simulink model "ObserverStatesPlusPert"  (R2022b)
settings: Solver=ode5  StartTime=0.0  StopTime=10  FixedStep=0.001  RelTol=1e-3
InitFcn:
  | ObsStatesPlusPertParameters
values from neighbouring files (symbols this model uses):
  A = 0.40648    [ObsStatesPlusPertParameters.m]
  a1 = e1/e2    (= 1.03595661896)    [ObsStatesPlusPertParameters.m]
  a2 = f2/e2    (= 0.828055342045)    [ObsStatesPlusPertParameters.m]
  a3 = f1/e2    (= 0.221523633506)    [ObsStatesPlusPertParameters.m]
  a4 = g2/e2    (= 0.768639508071)    [ObsStatesPlusPertParameters.m]
  a5 = g1/e2    (= 0.205628546835)    [ObsStatesPlusPertParameters.m]
  ax = 10.2    [ObsStatesPlusPertParameters.m]
  B = 0.40648    [ObsStatesPlusPertParameters.m]
  baralpha1 = 8    [ObsStatesPlusPertParameters.m]
  barbeta = 12.5    [ObsStatesPlusPertParameters.m]
  C = [1 , 0]    [ObsStatesPlusPertParameters.m]
  Cbar = [1, 0, 0]    [ObsStatesPlusPertParameters.m]
  G = 0.00833    [ObsStatesPlusPertParameters.m]
  Gamma = [ -a1, -a5 ... (first row only)    [ObsStatesPlusPertParameters.m]
  Gamma_bar = [    0,    ax,   0 ... (first row only)    [ObsStatesPlusPertParameters.m]
  k1 = 120    [ObsStatesPlusPertParameters.m]
  k1_pi = 20    [ObsStatesPlusPertParameters.m]
  k2 = 100    [ObsStatesPlusPertParameters.m]
  k2_pi = 1.3    [ObsStatesPlusPertParameters.m]
  kappa = 0.09    [ObsStatesPlusPertParameters.m]
  kobs = lobs/2 - (theta^3)/(2*ax)    (= 66.5945098039)    [ObsStatesPlusPertParameters.m]
  l = 0.65    [ObsStatesPlusPertParameters.m]
  L_b = 15    [ObsStatesPlusPertParameters.m]
  L_p = 7    [ObsStatesPlusPertParameters.m]
  M_b = 16    [ObsStatesPlusPertParameters.m]
  M_p = 7.1    [ObsStatesPlusPertParameters.m]
  omega = 1    [ObsStatesPlusPertParameters.m]
  Sinv = [    3*theta                            ,    3*((theta^2)/(ax))                     ,   (1/(ax))*(theta^3 + 2*kobs*ax) ... (first row only)    [ObsStatesPlusPertParameters.m]
settings Model: Creator=CIO  LastModifiedBy=gerar

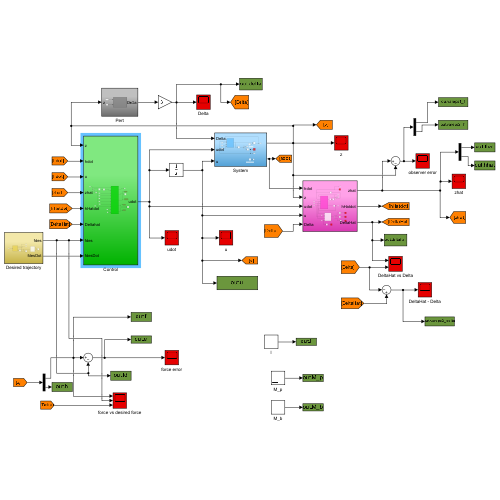
[thumbnail: Simulink's stored preview of the top-level diagram]
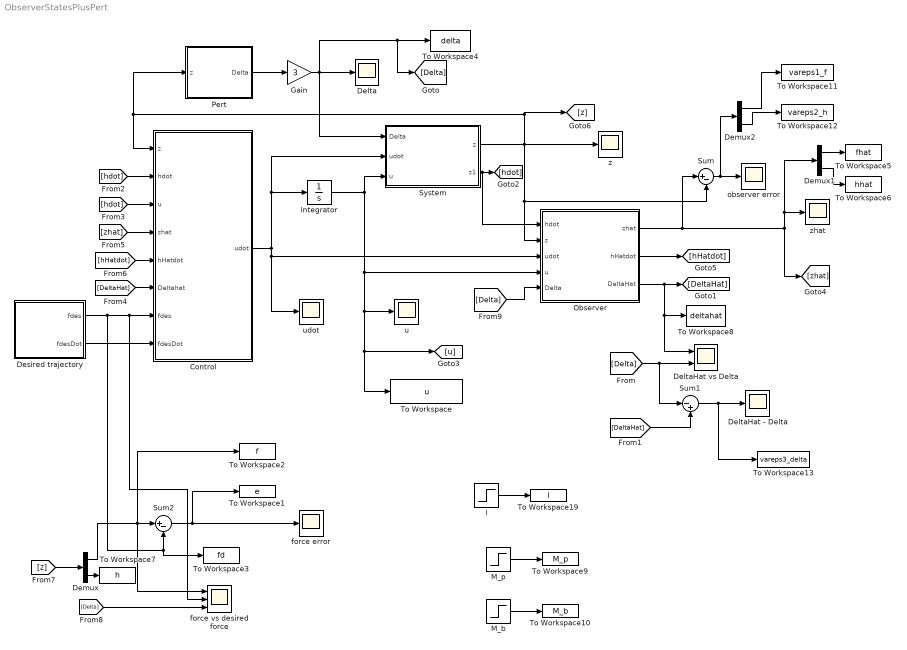
== system ObserverStatesPlusPert ==
  Control : Subsystem
  Delta : Scope
  DeltaHat - Delta : Scope
  DeltaHat vs Delta : Scope  NumInputPorts=2
  Demux : Demux  Outputs=2
  Demux1 : Demux  Outputs=2
  Demux2 : Demux  Outputs=2
  Desired trajectory : Subsystem
  Gain : Gain  Gain=3
  Integrator : Integrator
  M_b : Step  Time=0  Before=M_b  After=M_b  SampleTime=0
  M_p : Step  Time=0  Before=M_p  After=M_p  SampleTime=0
  Observer : Subsystem
  Pert : Subsystem
  Sum : Sum  Inputs=|+-
  Sum1 : Sum  Inputs=|-+
  Sum2 : Sum  Inputs=|+-
  System : Subsystem
  To Workspace : ToWorkspace  VariableName=u  SaveFormat=Timeseries  SampleTime=-1
  To Workspace1 : ToWorkspace  VariableName=e  SaveFormat=Timeseries  SampleTime=-1
  To Workspace10 : ToWorkspace  VariableName=M_b  SaveFormat=Timeseries  SampleTime=-1
  To Workspace11 : ToWorkspace  VariableName=vareps1_f  SaveFormat=Timeseries  SampleTime=-1
  To Workspace12 : ToWorkspace  VariableName=vareps2_h  SaveFormat=Timeseries  SampleTime=-1
  To Workspace13 : ToWorkspace  VariableName=vareps3_delta  SaveFormat=Timeseries  SampleTime=-1
  To Workspace19 : ToWorkspace  VariableName=l  SaveFormat=Timeseries  SampleTime=-1
  To Workspace2 : ToWorkspace  VariableName=f  SaveFormat=Timeseries  SampleTime=-1
  To Workspace3 : ToWorkspace  VariableName=fd  SaveFormat=Timeseries  SampleTime=-1
  To Workspace4 : ToWorkspace  VariableName=delta  SaveFormat=Timeseries  SampleTime=-1
  To Workspace5 : ToWorkspace  VariableName=fhat  SaveFormat=Timeseries  SampleTime=-1
  To Workspace6 : ToWorkspace  VariableName=hhat  SaveFormat=Timeseries  SampleTime=-1
  To Workspace7 : ToWorkspace  VariableName=h  SaveFormat=Timeseries  SampleTime=-1
  To Workspace8 : ToWorkspace  VariableName=deltahat  SaveFormat=Timeseries  SampleTime=-1
  To Workspace9 : ToWorkspace  VariableName=M_p  SaveFormat=Timeseries  SampleTime=-1
  force error : Scope
  force vs desired force : Scope  NumInputPorts=3
  l : Step  Time=0  Before=l  After=l  SampleTime=0
  observer error : Scope
  u : Scope
  udot : Scope
  z : Scope
  zhat : Scope
  wires:
  Control/1(udot) -> udot/1, Observer/3(udot), System/2(udot), Integrator/1
  System/1(z) -> Sum/2, Observer/2(z), z/1, [z], Pert/1(z), Control/1(z)
  Observer/1(zhat) -> [zhat], Demux1/1, zhat/1, Sum/1
  Sum/1 -> Demux2/1, observer error/1
  Pert/1(Delta) -> Gain/1
  Gain/1 -> To Workspace4/1, [Delta], Delta/1, System/1(Delta)
  Observer/3(DeltaHat) -> To Workspace8/1, DeltaHat vs Delta/1, [DeltaHat]
  [Delta] -> Sum1/1, DeltaHat vs Delta/2
  [DeltaHat] -> Sum1/2
  Sum1/1 -> To Workspace13/1, DeltaHat - Delta/1
  System/2(z1) -> Observer/1(hdot), [hdot]
  [hdot] -> Control/2(hdot)
  [hdot] -> Control/3(u)
  Integrator/1 -> System/3(u), To Workspace/1, [u], u/1, Observer/4(u)
  [DeltaHat] -> Control/6(Deltahat)
  [zhat] -> Control/4(zhat)
  Observer/2(hHatdot) -> [hHatdot]
  [hHatdot] -> Control/5(hHatdot)
  Desired trajectory/1(fdes) -> Control/7(fdes), force vs desired force/2, Sum2/2, To Workspace3/1
  Desired trajectory/2(fdesDot) -> Control/8(fdesDot)
  Sum2/1 -> To Workspace1/1, force error/1
  [z] -> Demux/1
  Demux/1 -> force vs desired force/1, Sum2/1, To Workspace2/1
  [Delta] -> force vs desired force/3
  Demux1/1 -> To Workspace5/1
  Demux1/2 -> To Workspace6/1
  Demux/2 -> To Workspace7/1
  l/1 -> To Workspace19/1
  M_p/1 -> To Workspace9/1
  M_b/1 -> To Workspace10/1
  [Delta] -> Observer/5(Delta)
  Demux2/1 -> To Workspace11/1
  Demux2/2 -> To Workspace12/1

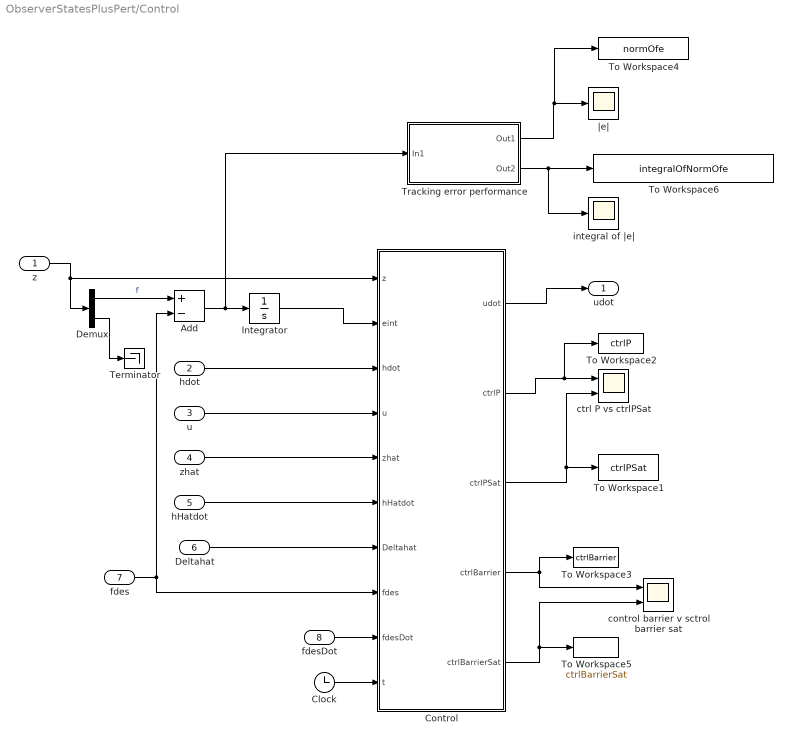
== system ObserverStatesPlusPert/Control ==
  z : Inport
  hdot : Inport  Port=2
  u : Inport  Port=3
  zhat : Inport  Port=4
  hHatdot : Inport  Port=5
  Deltahat : Inport  Port=6
  fdes : Inport  Port=7
  fdesDot : Inport  Port=8
  Add : Sum  Inputs=+-
  Clock : Clock
  Control : MATLAB Function  TreatAsAtomicUnit=on
  Demux : Demux  Outputs=2
  Integrator : Integrator
  Terminator : Terminator
  To Workspace1 : ToWorkspace  VariableName=ctrlPSat  SaveFormat=Timeseries  SampleTime=-1
  To Workspace2 : ToWorkspace  VariableName=ctrlP  SaveFormat=Timeseries  SampleTime=-1
  To Workspace3 : ToWorkspace  VariableName=ctrlBarrier  SaveFormat=Timeseries  SampleTime=-1
  To Workspace4 : ToWorkspace  VariableName=normOfe  SaveFormat=Timeseries  SampleTime=-1
  To Workspace5 : ToWorkspace  VariableName=ctrlBarrierSat  SaveFormat=Timeseries  SampleTime=-1
  To Workspace6 : ToWorkspace  VariableName=integralOfNormOfe  SaveFormat=Timeseries  SampleTime=-1
  Tracking error performance : Subsystem
  control barrier v sctrol barrier sat : Scope  NumInputPorts=2
  ctrl P vs ctrlPSat : Scope  NumInputPorts=2
  integral of |e| : Scope
  |e| : Scope
  udot : Outport
  wires:
  z/1 -> Demux/1, Control/1(z)
  Clock/1 -> Control/10(t)
  hdot/1 -> Control/3(hdot)
  u/1 -> Control/4(u)
  Deltahat/1 -> Control/7(Deltahat)
  zhat/1 -> Control/5(zhat)
  hHatdot/1 -> Control/6(hHatdot)
  Control/1(udot) -> udot/1
  fdes/1 -> Add/2, Control/8(fdes)
  fdesDot/1 -> Control/9(fdesDot)
  Control/4(ctrlBarrier) -> To Workspace3/1, control barrier v sctrol barrier sat/1
  Control/2(ctrlP) -> To Workspace2/1, ctrl P vs ctrlPSat/1
  Control/3(ctrlPSat) -> ctrl P vs ctrlPSat/2, To Workspace1/1
  Control/5(ctrlBarrierSat) -> control barrier v sctrol barrier sat/2, To Workspace5/1
  Demux/2 -> Terminator/1
  Demux/1 -> Add/1  "f"
  Add/1 -> Tracking error performance/1(In1), Integrator/1
  Integrator/1 -> Control/2(eint)
  Tracking error performance/1(Out1) -> To Workspace4/1, |e|/1
  Tracking error performance/2(Out2) -> integral of |e|/1, To Workspace6/1

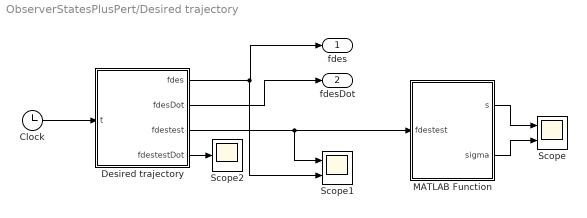
== system ObserverStatesPlusPert/Desired trajectory ==
  Clock : Clock
  Desired trajectory : MATLAB Function  TreatAsAtomicUnit=on
  MATLAB Function : MATLAB Function  TreatAsAtomicUnit=on
  Scope : Scope  NumInputPorts=2
  Scope1 : Scope  NumInputPorts=2
  Scope2 : Scope
  fdes : Outport
  fdesDot : Outport  Port=2
  wires:
  Clock/1 -> Desired trajectory/1(t)
  Desired trajectory/1(fdes) -> Scope1/2, fdes/1
  Desired trajectory/2(fdesDot) -> fdesDot/1
  MATLAB Function/1(s) -> Scope/1
  MATLAB Function/2(sigma) -> Scope/2
  Desired trajectory/3(fdestest) -> Scope1/1, MATLAB Function/1(fdestest)
  Desired trajectory/4(fdestestDot) -> Scope2/1

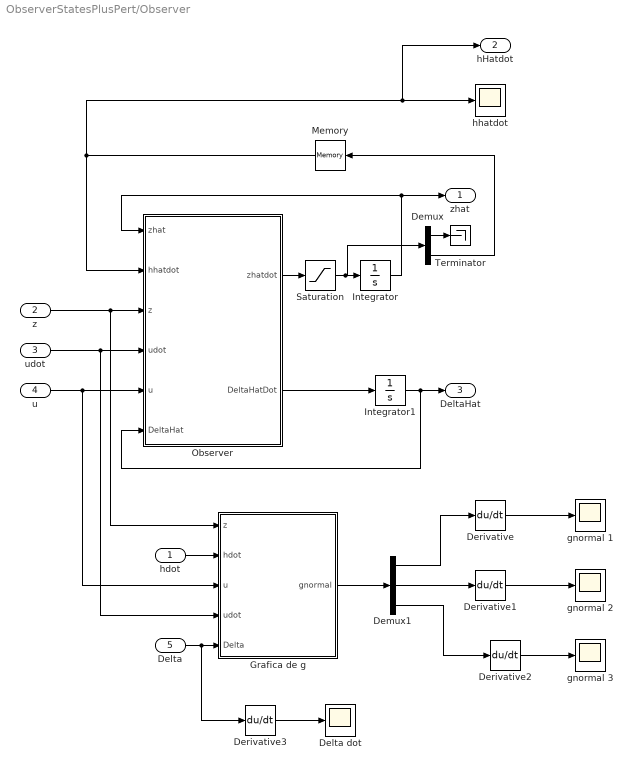
== system ObserverStatesPlusPert/Observer ==
  hdot : Inport
  z : Inport  Port=2
  udot : Inport  Port=3
  u : Inport  Port=4
  Delta : Inport  Port=5
  Delta dot : Scope
  Demux : Demux  Outputs=2
  Demux1 : Demux  Outputs=3
  Derivative{,1..3} (4 alike) : Derivative
  Grafica de g : MATLAB Function  TreatAsAtomicUnit=on
  Integrator : Integrator  InitialCondition=[0;0]
  Integrator1 : Integrator
  Memory : Memory
  Observer : MATLAB Function  TreatAsAtomicUnit=on
  Saturation : Saturate  UpperLimit=100  LowerLimit=-100
  Terminator : Terminator
  gnormal 1 : Scope
  gnormal 2 : Scope
  gnormal 3 : Scope
  hhatdot : Scope
  zhat : Outport
  hHatdot : Outport  Port=2
  DeltaHat : Outport  Port=3
  wires:
  Integrator/1 -> zhat/1, Observer/1(zhat)
  z/1 -> Grafica de g/1(z), Observer/3(z)
  udot/1 -> Grafica de g/4(udot), Observer/4(udot)
  u/1 -> Grafica de g/3(u), Observer/5(u)
  Demux/1 -> Terminator/1
  Demux/2 -> Memory/1
  Memory/1 -> hhatdot/1, hHatdot/1, Observer/2(hhatdot)
  Integrator1/1 -> DeltaHat/1, Observer/6(DeltaHat)
  Observer/1(zhatdot) -> Saturation/1
  Saturation/1 -> Integrator/1, Demux/1
  Observer/2(DeltaHatDot) -> Integrator1/1
  hdot/1 -> Grafica de g/2(hdot)
  Delta/1 -> Derivative3/1, Grafica de g/5(Delta)
  Grafica de g/1(gnormal) -> Demux1/1
  Demux1/1 -> Derivative/1
  Demux1/3 -> Derivative2/1
  Demux1/2 -> Derivative1/1
  Derivative/1 -> gnormal 1/1
  Derivative1/1 -> gnormal 2/1
  Derivative2/1 -> gnormal 3/1
  Derivative3/1 -> Delta dot/1

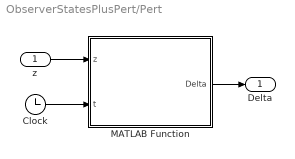
== system ObserverStatesPlusPert/Pert ==
  z : Inport
  Clock : Clock
  MATLAB Function : MATLAB Function  TreatAsAtomicUnit=on
  Delta : Outport
  wires:
  Clock/1 -> MATLAB Function/2(t)
  z/1 -> MATLAB Function/1(z)
  MATLAB Function/1(Delta) -> Delta/1

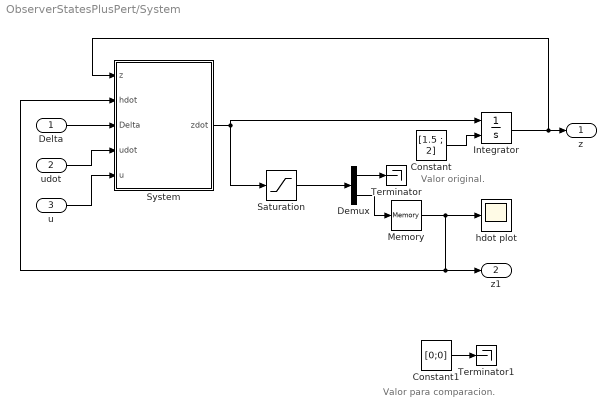
== system ObserverStatesPlusPert/System ==
  note: Valor para comparacion.
  note: Valor original.
  Delta : Inport
  udot : Inport  Port=2
  u : Inport  Port=3
  Constant : Constant  Value=[1.5 ; 2]
  Constant1 : Constant  Value=[0;0]
  Demux : Demux  Outputs=2
  Integrator : Integrator  InitialConditionSource=external  InitialCondition=[1.5;2]
  Memory : Memory
  Saturation : Saturate  UpperLimit=100  LowerLimit=-100
  System : MATLAB Function  TreatAsAtomicUnit=on
  Terminator : Terminator
  Terminator1 : Terminator
  hdot plot : Scope
  z : Outport
  z1 : Outport  Port=2
  wires:
  Integrator/1 -> System/1(z), z/1
  udot/1 -> System/4(udot)
  u/1 -> System/5(u)
  Demux/1 -> Terminator/1
  Demux/2 -> Memory/1
  Memory/1 -> hdot plot/1, z1/1, System/2(hdot)
  Delta/1 -> System/3(Delta)
  System/1(zdot) -> Saturation/1, Integrator/1
  Saturation/1 -> Demux/1
  Constant/1 -> Integrator/2
  Constant1/1 -> Terminator1/1

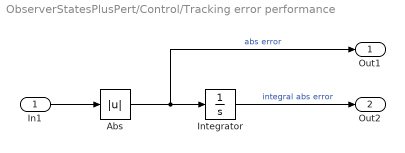
== system ObserverStatesPlusPert/Control/Tracking error performance ==
  In1 : Inport
  Abs : Abs  SaturateOnIntegerOverflow=off
  Integrator : Integrator
  Out1 : Outport
  Out2 : Outport  Port=2
  wires:
  In1/1 -> Abs/1
  Abs/1 -> Integrator/1, Out1/1  "abs error"
  Integrator/1 -> Out2/1  "integral abs error"

== matlab function ObserverStatesPlusPert/Pert/MATLAB Function ==
  data: z input; t input; Delta output
function Delta = pert(z, t)
  
% original
% Delta = 2*cos(t) + 1.0;

% agresive
Delta = 2*cos(t) + 1.0 + 2*rectpuls(t-6,1) - 2*rectpuls(t-7,1);

% ancient
% Delta = 0.5*cos(0.1*t);

== matlab function ObserverStatesPlusPert/Desired trajectory/Desired trajectory ==
  data: t input; fdes output; fdesDot output; fdestest output; omega parameter; kappa parameter; fdestestDot output
function [fdes, fdesDot, fdestest, fdestestDot] = des(t, omega, kappa)

%fdes = 2*sin(t) + 2;
%fdesDot = 2*cos(t);
%fdestest = 10*sin(t);




% Squdel function


sqd_s = 1 * (( sin(omega*t) )/( sqrt(  (sin(omega*t))^2 + kappa^2*(cos(omega*t))^2  ) ) + 1 );
sqd_sDot = 1 * ( (  kappa^2*omega*cos(omega*t) )/(  (1+kappa^2)/(2) - ((1-kappa^2)/(2))*cos(2*omega*t)  )^(3/2) ) ;

sqd_c = 1 * (( cos(omega*t) )/( sqrt(  kappa^2*(sin(omega*t))^2 + (cos(omega*t))^2  ) ) + 1 );
sqd_cDot = - 1 * ( (  kappa^2*omega*sin(omega*t) )/(  (cos(omega*t))^2 + kappa^2*(sin(omega*t))^2  )^(3/2) ) ;



fdestest = sqd_s;
fdestestDot = sqd_sDot;



% asignement
fdes = sqd_c;
fdesDot = sqd_cDot;

% %% Para comparacion con trabajos de Micky [CAMBIAR t = 40]
% fdes = 20e-03;
% fdesDot = 0;

== matlab function ObserverStatesPlusPert/Desired trajectory/MATLAB Function ==
  data: fdestest input; s output; sigma output
function [s, sigma] = sat(fdestest)

L_ij = 1;
M_ij = 1.5;
a = (pi)/(2*(M_ij - L_ij));
s = fdestest;

if s > L_ij
    sigma = tanh(a*(s - L_ij))/(a) + L_ij;
elseif abs(s) <= L_ij
    sigma = s;
elseif s < (-L_ij)
    sigma = tanh(a*(s + L_ij))/(a) - L_ij;
else
    sigma = 0;
    %eml.extrinsic('fprintf')
    %fprintf('None of the values are matching\n');
end

== matlab function ObserverStatesPlusPert/Observer/Grafica de g ==
  data: z input; hdot input; u input; udot input; Delta input; gnormal output; a1 parameter; a3 parameter; a4 parameter; a5 parameter; kobs parameter; ax parameter; B parameter; G parameter
function gnormal = fcn(z, hdot, u, udot, Delta, a1, a3, a4, a5, kobs, ax, B, G)

f = z(1,1);
h = z(2,1);

% Solo para propositos de graficar, asumiendo que conocemos todo.
gnormal = [- a1*f  + a3*u - a4*hdot - a5*h + Delta - ax*h ;
           - B*abs(udot)*h - G*udot*abs(h) - Delta          ;
           -kobs*f                                         ]; % just for plot, not used here

== matlab function ObserverStatesPlusPert/Control/Control ==
  data: z input; eint input; hdot input; u input; zhat input; hHatdot input; Deltahat input; fdes input; fdesDot input; udot output; t input; a1 parameter; a2 parameter; a3 parameter; a4 parameter; a5 parameter; ctrlP output; ctrlPSat output; ctrlBarrier output; ctrlBarrierSat output; l parameter; k1 parameter; k2 parameter; L_p parameter; M_p parameter; L_b parameter; M_b parameter; k1_pi parameter; k2_pi parameter; baralpha1 parameter; barbeta parameter
function [udot, ctrlP, ctrlPSat, ctrlBarrier, ctrlBarrierSat] = ctrl(z, eint, hdot, u, zhat, hHatdot, Deltahat, fdes, fdesDot, t, a1, a2, a3, a4, a5, l, k1, k2, L_p, M_p, L_b, M_b, k1_pi, k2_pi, baralpha1, barbeta)

f    = z(1,1);          h = z(2,1);
fhat = zhat(1,1);       hhat = zhat(2,1);

err = f - fdes;    % tracking error
% hdothat = zhatdot(2,1); %Este me esta causando errores

%%%%%%%%%%%%%%%%%%%%%%%% saturacion 
ctrlP = - (k1*err)*(l^2 - err^2); % - 120*err; ; - 60*err;
aP = (pi)/(2*(M_p - L_p));
sp = ctrlP;

if sp > L_p
    sigmaP = tanh(aP*(sp - L_p))/(aP) + L_p;
elseif abs(sp) <= L_p
    sigmaP = sp;
elseif sp < (-L_p)
    sigmaP = tanh(aP*(sp + L_p))/(aP) - L_p;
else
    sigmaP = 0;
    %eml.extrinsic('fprintf')
    %fprintf('None of the values are matching\n');
end


ctrlBarrier = - k2*err/(l^2 - err^2); %- 100*err/(l^2 - err^2) - 80*err/(l^2 - err^2);
aB = (pi)/(2*(M_b - L_b));
sb = ctrlBarrier;

if sb > L_b
    sigmaB = tanh(aB*(sb - L_b))/(aB) + L_b;
elseif abs(sb) <= L_b
    sigmaB = sb;
elseif sb < (-L_b)
    sigmaB = tanh(aB*(sb + L_b))/(aB) - L_b;
else
    sigmaB = 0;
    %eml.extrinsic('fprintf')
    %fprintf('None of the values are matching\n');
end

ctrlPSat = sigmaP;
ctrlBarrierSat = sigmaB;
%%%%%%%%%%%%%%%%%%%%%%%% saturacion

%% El de este paper
udot = (1/a2)*( a1*f + a5*hhat - a3*u + a4*hHatdot + ctrlPSat + ctrlBarrierSat + fdesDot - Deltahat  ) ;

% %% PI
% udot_PI = (1/a2)*( a1*f + a5*hhat - a3*u + a4*hHatdot - k1_pi*err - k2_pi*eint + fdesDot ) ;
% udot = udot_PI;

% %% SMC
% rho_smc = err + baralpha1*eint;
% udot_SMC = (1/a2)*( a1*f + a5*hhat - a3*u + a4*hHatdot - barbeta*sign(rho_smc) + fdesDot ) ;
% udot = udot_SMC;

== matlab function ObserverStatesPlusPert/System/System ==
  data: z input; hdot input; Delta input; udot input; u input; zdot output; Gamma parameter; a2 parameter; A parameter; B parameter; G parameter; a3 parameter; a4 parameter
function zdot = fcn(z, hdot, Delta, udot, u, Gamma, a2, A, B, G, a3, a4)

f = z(1,1);
h = z(2,1);

g_ = [ a2*udot + a3*u - a4*hdot               ;
       A*udot - B*abs(udot)*h - G*udot*abs(h)]; 
     

zdot = Gamma*z + g_ + [1; 0]*Delta;

== matlab function ObserverStatesPlusPert/Observer/Observer ==
  data: zhat input; hhatdot input; zhatdot output; z input; udot input; u input; DeltaHat input; A parameter; B parameter; G parameter; Sinv parameter; a2 parameter; C parameter; a3 parameter; a4 parameter; DeltaHatDot output; a1 parameter; a5 parameter; kobs parameter; Cbar parameter; Gamma_bar parameter; ax parameter
function [zhatdot, DeltaHatDot] = obs(zhat, hhatdot, z, udot, u, DeltaHat, A, B, G, Sinv, a2, C, a3, a4, a1, a5, kobs, Cbar, Gamma_bar, ax)


fhat = zhat(1,1);
hhat = zhat(2,1);
e = zhat - z;

g_hat = [ a2*udot + a3*u - a4*hhatdot                  ;    %tal cual lo tiene el sistema
          A*udot - B*abs(udot)*hhat - G*udot*abs(hhat)]; 

% Este reacomodo solo se hace para el analisis, pero realmente queda como
% una copia del sistema; se estan sumando y restando terminos

g_hatBar = [g_hat ;   
              0   ] ...
                        +  [ - a1*fhat - ax*hhat - a5*hhat        ;
                             - DeltaHat                           ; 
                             - kobs*fhat                         ];

Xhat = [ zhat    ;
        DeltaHat ];

Xhatdot = Gamma_bar*Xhat + g_hatBar + [1;0;0]*DeltaHat - Sinv*Cbar'*(C*e);



zhatdot     = [ Xhatdot(1,1);
                Xhatdot(2,1)];
DeltaHatDot =   Xhatdot(3,1);





















% New observer:
% Cbar = [1, 0, 0];
% Gamma_bar = [-a1, -a5,  1 ;
%               0,   0,  0 ;
%               0,   0,  0 ];
% 
% 
% Gamma_bar = [  0,   1,  0 ;
%                0,   0,  1 ;
%                0,   0,  0 ];
% 
% g_hatBar = [ g_hat ;
%               0    ];
% 
% Q = [ 3*theta   ,   3*theta^2,   theta^3   ;
%       3*theta^2 ,   5*theta^3,   2*theta^4 ;
%       theta^3   ,   2*theta^4,   theta^5   ]; %ajustandole la primera columna sale = [30*theta; 3*theta^2; 30*theta^3 ] y theta = 3;
% 
% Xhat = [ zhat    ;
%         DeltaHat ];
% 
% Xhatdot = Gamma_bar*Xhat + g_hatBar - Q*Cbar'*e(1,1);
% 
% 
% 
% zhatdot     = [ Xhatdot(1,1);
%                 Xhatdot(2,1)];
% DeltaHatDot =   Xhatdot(3,1);



% con este funciono:
% k = -(1/(2*a5))*(theta^3 - 450);
% DeltaHatDot = -((1/a5^2)*(theta^3*a5 + 2*k*a5^2))*(C*e);  %- 120*(C*e) -(1/a5^2)*(theta^3*a5 + 2*k*a5^2)*(C*e); - 120*(C*e);
